simulink model "arithmetic2023"  (R2025a)
settings: Solver=FixedStepAuto  StartTime=0.0  StopTime=15  FixedStep=0.00001  MaxStep=0.001  RelTol=1e-3
values from neighbouring files (symbols this model uses):
  A = 1.5    [data2023.sldd]    (also in lqr_K.m = [0 1 0 0)
  drone_r0 = 0.0 100.0    [data.sldd]    (also in data2023.sldd = 0.0 60.0)
  Fx = 600.0    [data.sldd]    (also in data2023.sldd)
  Fy = 800.0    [data.sldd]    (also in data2023.sldd)
  g = 10.0    [data.sldd]    (also in data2023.sldd = 9.81)
  K = 3.1623 -0.0 2.7064 0.0 -0.0 3.1623 -0.0 2.7064    [data2023.sldd]    (also in lqr_K.m = lqr(A, B, Q, R))
  ma = 20.0    [data.sldd]    (also in data2023.sldd)
  mb = 50.0    [data.sldd]    (also in data2023.sldd)
  T0 = 20.0    [data.sldd]    (also in data2023.sldd)
settings Model: DataDictionary=data2023.sldd  Creator=MangoJuice  LastModifiedBy=MangoJuice

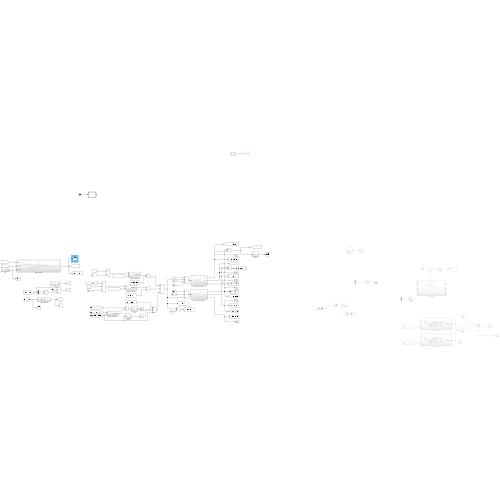
[thumbnail: Simulink's stored preview of the top-level diagram]
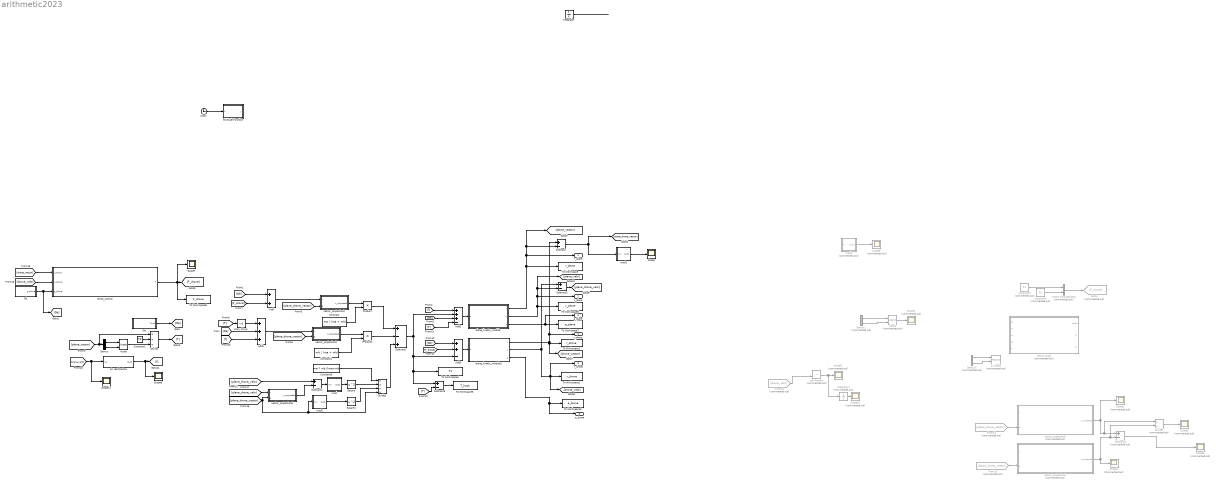
== system arithmetic2023 ==
  Add : Sum
  Add1 : Sum  Inputs=+++
  Add2 : Sum  Inputs=+++-
  Add3 : Sum  Inputs=++-
  Atan2 : Trigonometry  Commented=on  Operator=atan2
  Clock : Clock
  Constant : Constant  Value=ma / (ma + mb)
  Constant1 : Constant  Value=mb / (ma + mb)
  Constant2 : Constant  Value=T0
  Constant3 : Constant  Commented=on  Value=Fx
  Constant4 : Constant  Commented=on  Value=Fy
  Constant5 : Constant  Value=ma * mb /(ma+mb)
  Demux : Demux  Outputs=2
  Demux1 : Demux  Commented=on  Outputs=2
  Demux3 : Demux  Commented=on  Outputs=2
  Divide : Product  Inputs=**/
  Divide1 : Product  Commented=on  Inputs=*/
  Divide2 : Product  Inputs=**/*
  Dot Product : DotProduct  Commented=on  OutDataTypeStr=Inherit: Inherit via internal rule
  From13 : From  Commented=on  GotoTag=plane_drone_vector
  From14 : From  Commented=on  GotoTag=plane_drone_vector
  From20 : From  Commented=on  GotoTag=drone_velo
  Ga : Subsystem
  Gb : Subsystem
  Goto4 : Goto  Commented=on  GotoTag=F_drone
  Hypot : Math  Operator=hypot
  Integrator : Integrator
  Integrator1 : Integrator  Commented=on
  MATLAB Function : MATLAB Function  TreatAsAtomicUnit=on  SystemSampleTime=0.1
  Product : Product
  Product1 : Product
  Scope{,6..7,11} (4 alike) : Scope
      Scope settings: ActiveDisplayYMinimum=21.853261118393789  ActiveDisplayYMaximum=40.402568271734616
      Scope11 settings: ActiveDisplayYMinimum=-28.733519725359326  ActiveDisplayYMaximum=28.020670582045391  DataLoggingVariableName=ScopeData11
      Scope6 settings: ActiveDisplayYMinimum=-1  ActiveDisplayYMaximum=1  DataLoggingVariableName=ScopeData6
      Scope7 settings: ActiveDisplayYMinimum=-4257.5776928327887  ActiveDisplayYMaximum=3270.59159962983  DataLoggingVariableName=ScopeData7
  Scope{1..5,8..10} (8 alike) : Scope  Commented=on
      Scope1 settings: ActiveDisplayYMinimum=-1.0944  ActiveDisplayYMaximum=6.4337
      Scope10 settings: ActiveDisplayYMinimum=-1854.0026966671489  ActiveDisplayYMaximum=1339.365502512725  DataLoggingVariableName=ScopeData10
      Scope2 settings: ActiveDisplayYMinimum=-1  ActiveDisplayYMaximum=1  DataLoggingVariableName=ScopeData2
      Scope3 settings: ActiveDisplayYMinimum=-1.274  ActiveDisplayYMaximum=0.99186  DataLoggingVariableName=ScopeData3
      Scope4 settings: ActiveDisplayYMinimum=-0.28044128715875616  ActiveDisplayYMaximum=1.7069968813063119  DataLoggingVariableName=ScopeData4
      Scope5 settings: ActiveDisplayYMinimum=-10.224  ActiveDisplayYMaximum=15.1156  DataLoggingVariableName=ScopeData5
      Scope8 settings: ActiveDisplayYMinimum=45.49151131182159  ActiveDisplayYMaximum=877.68274656123344  DataLoggingVariableName=ScopeData8
      Scope9 settings: ActiveDisplayYMinimum=-1254.7088806848469  ActiveDisplayYMaximum=461.43323334308008  DataLoggingVariableName=ScopeData9
  Square : Math  Operator=square
  Square1 : Math  Operator=square
  Subtract{,3..5} (4 alike) : Sum  Inputs=+-
  Subtract1 : Sum  Inputs=+-+
  Subtract2 : Sum  Commented=on  Inputs=+-
  To Workspace : ToWorkspace  VariableName=r_plane  SaveFormat=Timeseries  SampleTime=0.05
  To Workspace1 : ToWorkspace  VariableName=r_drone  SaveFormat=Timeseries  SampleTime=0.05
  To Workspace2 : ToWorkspace  VariableName=v_drone  SaveFormat=Timeseries  SampleTime=0.05
  To Workspace3 : ToWorkspace  VariableName=a_drone  SaveFormat=Timeseries  SampleTime=0.05
  To Workspace4 : ToWorkspace  VariableName=T1  SaveFormat=Timeseries  SampleTime=0.05
  To Workspace5 : ToWorkspace  VariableName=T_hook  SaveFormat=Timeseries  SampleTime=0.05
  To Workspace6 : ToWorkspace  VariableName=v_plane  SaveFormat=Timeseries  SampleTime=0.05
  To Workspace7 : ToWorkspace  VariableName=a_plane  SaveFormat=Timeseries  SampleTime=0.05
  To Workspace8 : ToWorkspace  VariableName=F_drone  SaveFormat=Timeseries  SampleTime=0.05
  Unary Minus : UnaryMinus
  Vector Concatenate1 : Concatenate  Commented=on
  XY Graph : Record  Commented=on  NumPorts=2.0  FileSettingsInternal="{\"entries\":[{\"content\":{\"excelSettings\":{\"content\":{},\"type\":\"Streamout.ExcelSettings\"},\"parquetSettings\":{\"content\":{},\"type\":\"Streamout.ParquetSettings\"}},\"type\":\"Streamout.FileSettingStorage\",\"uuid\":\"\"}],\"packageUris\":[\"http:\\/\\/schema.mathworks.com\\/mf0\\/streamout_blocks\\/R2020a\"],\"version\":\"1.0\"}"  FrameSettings=[0, 0]  Layout=[1 1]  SignalsInternal="{\"entries\":[{\"content\":{\"signals\":[{\"content\":{\"blockPath\":[],\"dimensions\":[1],\"domain\":\"\",\"lineColor\":\"#a2142f\",\"plots\":[ 1 ],\"port\":1,\"signalID\":1,\"signalName\":\"Demux3:1\"},\"type\":\"RecordBlkView.Signal\",\"uuid\":\"\"},{\"content\":{\"blockPath\":[],\"dimensions\":[1],\"domain\":\"\",\"lineColor\":\"#139fff\",\"plots\":[ 1 ],\"port\":2,\"signalID\":2,\"signalName\":\"Demux3:2\"},\"type\":\"RecordBlkView.Signal\",\"uuid\":\"\"}]},\"type\":\"RecordBlkView.InputSignals\",\"uuid\":\"\"}],\"packageUris\":[\"http:\\/\\/schema.mathworks.com\\/mf0\\/streamout_blocks\\/R2020a\"],\"version\":\"1.0\"}"  VisualizationBindings="{\"xyplotplugin\":{\"info\":[{\"series\":[{\"bindingParametersList\":[{\"parameter\":\"X-Axis\",\"signalID\":1,\"signalName\":\"Demux3:1\"},{\"parameter\":\"Y-Axis\",\"signalID\":2,\"signalName\":\"Demux3:2\"}],\"seriesID\":0}],\"subplotID\":1}]}}"  CompatibilityTag=XY
  air resistantce : Subsystem
  drone_control : Subsystem
  drone_kinetic_module1 : Subsystem
  mod : Subsystem
  mod1 : Subsystem
  mod2 : Subsystem
  mod3 : Subsystem  Commented=on
  plane_kinetic_module : Subsystem
  vector-angle : Subsystem  Commented=on
  vector_projection2 : Subsystem
  vector_projection3 : Subsystem
  vector_projection4 : Subsystem  Commented=on
  vector_projection5 : Subsystem  Commented=on
  vector_projection6 : Subsystem
  r_plane : Outport
  v_plane : Outport  Port=2
  a_plane : Outport  Port=3
  r_drone : Outport  Port=4
  v_drone : Outport  Port=5
  a_drone : Outport  Port=6
  wires:
  Integrator/1 -> ?
  Ga/1(Out1) -> [Ga]
  Gb/1(g_drone) -> [Gb], drone_control/3(g_drone)
  Subtract/1 -> mod1/1(In1), [plane_drone_vector]
  Hypot/1 -> Divide/3
  [plane_vector] -> Divide/1, Demux/1
  Demux/2 -> Hypot/2
  Demux/1 -> Hypot/1
  Constant2/1 -> Divide/2
  Vector Concatenate1/1 -> Goto4/1
  Constant3/1 -> Vector Concatenate1/1
  Constant4/1 -> Vector Concatenate1/2
  [plane_drone_vector] -> vector_projection2/2(e)
  [plane_drone_vector] -> vector_projection3/2(e)
  [Gb] -> Add/1
  Product/1 -> Subtract1/1
  Product1/1 -> Subtract1/2
  Constant/1 -> Product/2
  Constant1/1 -> Product1/2
  Subtract1/1 -> Add2/2, Subtract5/1, To Workspace4/1, Add3/3
  Add2/1 -> plane_kinetic_module/1(F)
  [Ga] -> Add2/3
  [T] -> Add2/4
  Add3/1 -> drone_kinetic_module1/1(F)
  [F_drone] -> Add3/2
  [Gb] -> Add3/1
  vector_projection5/1(x_projected) -> Scope1/1, Divide1/1, Subtract2/1
  vector_projection4/1(x_projected) -> Scope2/1, Divide1/2, Subtract2/2
  From14/1 -> vector_projection5/2(e)
  From13/1 -> vector_projection4/2(e)
  Demux3/2 -> XY Graph/2
  Demux3/1 -> XY Graph/1
  Divide/1 -> [T]
  [T] -> Unary Minus/1
  Subtract2/1 -> Scope5/1
  Divide1/1 -> Scope3/1
  Subtract3/1 -> [plane_drone_velo]
  [plane_drone_velo] -> vector_projection6/1(x)
  vector_projection6/1(x_projected) -> Subtract4/2
  [plane_drone_velo] -> Subtract4/1
  Subtract4/1 -> mod/1(In1)
  mod/1(Out1) -> Square/1
  mod2/1(Out1) -> Square1/1
  [plane_drone_vector] -> vector_projection6/2(e), Divide2/4, mod2/1(In1)
  Square/1 -> Divide2/2
  Square1/1 -> Divide2/3
  Divide2/1 -> Subtract1/3
  Constant5/1 -> Divide2/1
  mod1/1(Out1) -> Scope/1
  Atan2/1 -> Scope4/1
  Demux1/1 -> Atan2/1
  Demux1/2 -> Atan2/2
  [drone_velo] -> drone_control/2(v_drone)
  [drone_vector] -> drone_control/1(r_drone)
  mod3/1(Out1) -> Scope8/1
  drone_control/1(F) -> To Workspace8/1, Scope7/1, [F_drone]
  From20/1 -> Dot Product/2
  Dot Product/1 -> Integrator1/1, Scope9/1
  Integrator1/1 -> Scope10/1
  Clock/1 -> MATLAB Function/1(t)
  [T] -> Subtract5/2
  Subtract5/1 -> To Workspace5/1
  drone_kinetic_module1/1(r) -> [drone_vector], To Workspace1/1, Subtract/1, r_drone/1
  drone_kinetic_module1/2(v) -> [drone_velo], v_drone/1, To Workspace2/1, Subtract3/1
  drone_kinetic_module1/3(a) -> a_drone/1, To Workspace3/1
  plane_kinetic_module/3(a) -> a_plane/1, To Workspace7/1
  plane_kinetic_module/2(v) -> [plane_velo], Subtract3/2, v_plane/1, To Workspace6/1
  plane_kinetic_module/1(r) -> [plane_vector], Subtract/2, r_plane/1, To Workspace/1
  [plane_velo] -> Scope11/1, air resistantce/1(In1)
  air resistantce/1(Out1) -> Scope6/1, [f]
  Unary Minus/1 -> Add1/1
  [Ga] -> Add1/2
  [f] -> Add1/3
  Add1/1 -> vector_projection3/1(x)
  vector_projection3/1(x_projected) -> Product1/1
  [F_drone] -> Add/2
  vector_projection2/1(x_projected) -> Product/1
  Add/1 -> vector_projection2/1(x)
  [f] -> Add2/1

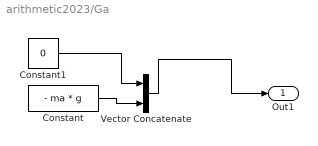
== system arithmetic2023/Ga ==
  Constant : Constant  Value=- ma * g  VectorParams1D=off
  Constant1 : Constant  Value=0
  Vector Concatenate : Concatenate
  Out1 : Outport
  wires:
  Constant1/1 -> Vector Concatenate/1
  Constant/1 -> Vector Concatenate/2
  Vector Concatenate/1 -> Out1/1

== system arithmetic2023/Gb ==
  Constant : Constant  Value=- mb * g  VectorParams1D=off
  Constant1 : Constant  Value=0
  Vector Concatenate : Concatenate
  g_drone : Outport
  wires:
  Vector Concatenate/1 -> g_drone/1
  Constant/1 -> Vector Concatenate/2
  Constant1/1 -> Vector Concatenate/1

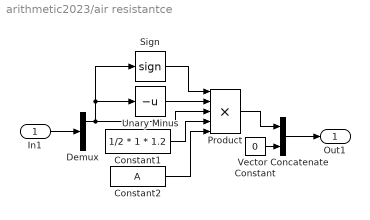
== system arithmetic2023/air resistantce ==
  In1 : Inport
  Constant : Constant  Value=0
  Constant1 : Constant  Value=1/2 * 1 * 1.2
  Constant2 : Constant  Value=A
  Demux : Demux  Outputs=2
  Product : Product  Inputs=5
  Sign : Signum
  Unary Minus : UnaryMinus
  Vector Concatenate : Concatenate
  Out1 : Outport
  wires:
  In1/1 -> Demux/1
  Demux/1 -> Product/3, Sign/1, Unary Minus/1
  Unary Minus/1 -> Product/2
  Constant1/1 -> Product/4
  Constant2/1 -> Product/5
  Product/1 -> Vector Concatenate/1
  Constant/1 -> Vector Concatenate/2
  Vector Concatenate/1 -> Out1/1
  Sign/1 -> Product/1

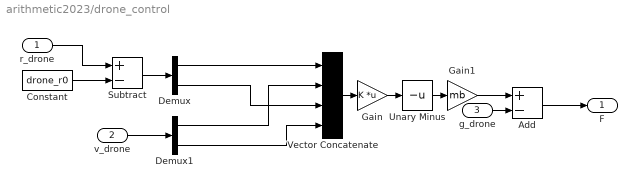
== system arithmetic2023/drone_control ==
  r_drone : Inport
  v_drone : Inport  Port=2
  g_drone : Inport  Port=3
  Add : Sum  Inputs=+-
  Constant : Constant  Value=drone_r0
  Demux : Demux  Outputs=2
  Demux1 : Demux  Outputs=2
  Gain : Gain  Gain=K  Multiplication=Matrix(K*u)
  Gain1 : Gain  Gain=mb
  Subtract : Sum  Inputs=+-
  Unary Minus : UnaryMinus
  Vector Concatenate : Concatenate  NumInputs=4
  F : Outport
  wires:
  Demux/1 -> Vector Concatenate/1
  Demux/2 -> Vector Concatenate/3
  v_drone/1 -> Demux1/1
  Demux1/2 -> Vector Concatenate/4
  Demux1/1 -> Vector Concatenate/2
  Vector Concatenate/1 -> Gain/1
  Unary Minus/1 -> Gain1/1
  Gain/1 -> Unary Minus/1
  Add/1 -> F/1
  Subtract/1 -> Demux/1
  r_drone/1 -> Subtract/1
  Constant/1 -> Subtract/2
  g_drone/1 -> Add/2
  Gain1/1 -> Add/1

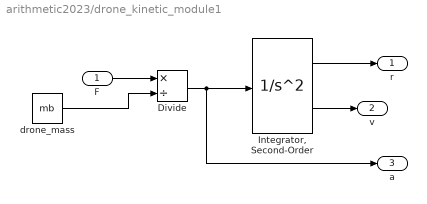
== system arithmetic2023/drone_kinetic_module1 ==
  F : Inport
  Divide : Product  Inputs=*/
  "Integrator, Second-Order" : SecondOrderIntegrator  ICX=drone_r0  ICDXDT=drone_v0
  drone_mass : Constant  Value=mb
  r : Outport
  v : Outport  Port=2
  a : Outport  Port=3
  wires:
  drone_mass/1 -> Divide/2
  "Integrator, Second-Order"/2 -> v/1
  "Integrator, Second-Order"/1 -> r/1
  Divide/1 -> a/1, "Integrator, Second-Order"/1
  F/1 -> Divide/1

== system arithmetic2023/mod ==
  In1 : Inport
  Demux4 : Demux  Outputs=2
  Hypot3 : Math  Operator=hypot
  Out1 : Outport
  wires:
  Demux4/1 -> Hypot3/1
  Demux4/2 -> Hypot3/2
  In1/1 -> Demux4/1
  Hypot3/1 -> Out1/1

== system arithmetic2023/mod1 ==
  In1 : Inport
  Demux4 : Demux  Outputs=2
  Hypot3 : Math  Operator=hypot
  Out1 : Outport
  wires:
  Demux4/1 -> Hypot3/1
  Demux4/2 -> Hypot3/2
  In1/1 -> Demux4/1
  Hypot3/1 -> Out1/1

== system arithmetic2023/mod2 ==
  In1 : Inport
  Demux4 : Demux  Outputs=2
  Hypot3 : Math  Operator=hypot
  Out1 : Outport
  wires:
  Hypot3/1 -> Out1/1
  In1/1 -> Demux4/1
  Demux4/2 -> Hypot3/2
  Demux4/1 -> Hypot3/1

== system arithmetic2023/mod3 ==
  F : Inport
  Demux4 : Demux  Outputs=2
  Hypot3 : Math  Operator=hypot
  Out1 : Outport
  wires:
  Hypot3/1 -> Out1/1
  F/1 -> Demux4/1
  Demux4/2 -> Hypot3/2
  Demux4/1 -> Hypot3/1

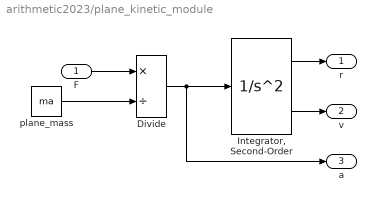
== system arithmetic2023/plane_kinetic_module ==
  F : Inport
  Divide : Product  Inputs=*/
  "Integrator, Second-Order" : SecondOrderIntegrator  ICX=plane_r0  ICDXDT=plane_v0
  plane_mass : Constant  Value=ma
  r : Outport
  v : Outport  Port=2
  a : Outport  Port=3
  wires:
  F/1 -> Divide/1
  Divide/1 -> "Integrator, Second-Order"/1, a/1
  "Integrator, Second-Order"/1 -> r/1
  "Integrator, Second-Order"/2 -> v/1
  plane_mass/1 -> Divide/2

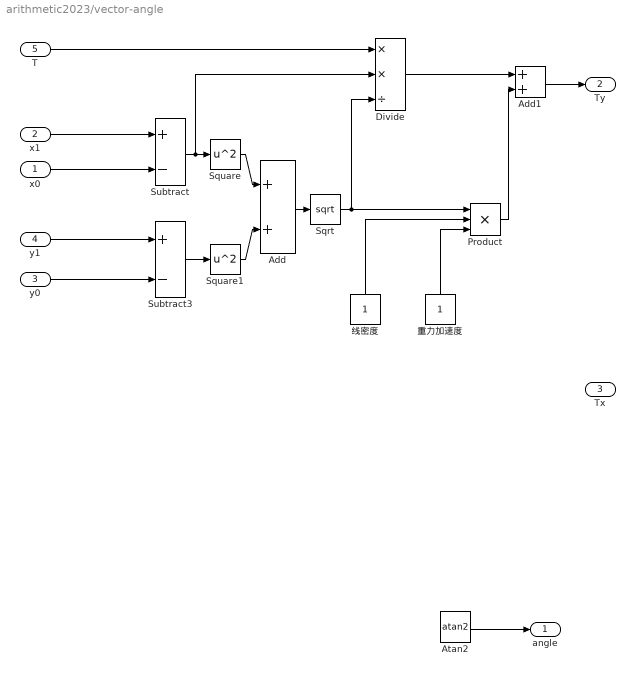
== system arithmetic2023/vector-angle ==
  x0 : Inport
  x1 : Inport  Port=2
  y0 : Inport  Port=3
  y1 : Inport  Port=4
  T : Inport  Port=5
  Add : Sum
  Add1 : Sum
  Atan2 : Trigonometry  Operator=atan2
  Divide : Product  Inputs=**/
  Product : Product  Inputs=3
  Sqrt : Sqrt
  Square : Math  Operator=square
  Square1 : Math  Operator=square
  Subtract : Sum  Inputs=+-
  Subtract3 : Sum  Inputs=+-
  线密度 : Constant
  重力加速度 : Constant
  angle : Outport
  Ty : Outport  Port=2
  Tx : Outport  Port=3
  wires:
  y0/1 -> Subtract3/2
  x1/1 -> Subtract/1
  Atan2/1 -> angle/1
  x0/1 -> Subtract/2
  y1/1 -> Subtract3/1
  Subtract/1 -> Divide/2, Square/1
  Subtract3/1 -> Square1/1
  Square/1 -> Add/1
  Square1/1 -> Add/2
  线密度/1 -> Product/2
  重力加速度/1 -> Product/3
  T/1 -> Divide/1
  Add/1 -> Sqrt/1
  Sqrt/1 -> Divide/3, Product/1
  Divide/1 -> Add1/1
  Product/1 -> Add1/2
  Add1/1 -> Ty/1

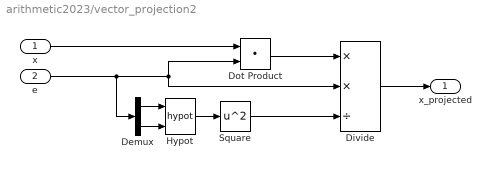
== system arithmetic2023/vector_projection2 ==
  x : Inport
  e : Inport  Port=2
  Demux : Demux  Outputs=2
  Divide : Product  Inputs=**/
  Dot Product : DotProduct  OutDataTypeStr=Inherit: Inherit via internal rule
  Hypot : Math  Operator=hypot
  Square : Math  Operator=square
  x_projected : Outport
  wires:
  x/1 -> Dot Product/1
  Divide/1 -> x_projected/1
  Hypot/1 -> Square/1
  e/1 -> Demux/1, Dot Product/2, Divide/2
  Demux/2 -> Hypot/2
  Demux/1 -> Hypot/1
  Square/1 -> Divide/3
  Dot Product/1 -> Divide/1

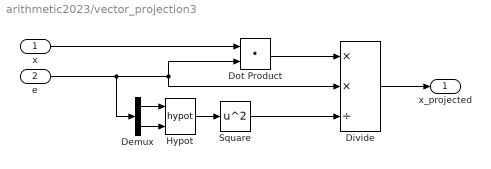
== system arithmetic2023/vector_projection3 ==
  x : Inport
  e : Inport  Port=2
  Demux : Demux  Outputs=2
  Divide : Product  Inputs=**/
  Dot Product : DotProduct  OutDataTypeStr=Inherit: Inherit via internal rule
  Hypot : Math  Operator=hypot
  Square : Math  Operator=square
  x_projected : Outport
  wires:
  Dot Product/1 -> Divide/1
  Square/1 -> Divide/3
  Demux/1 -> Hypot/1
  Demux/2 -> Hypot/2
  e/1 -> Divide/2, Dot Product/2, Demux/1
  Hypot/1 -> Square/1
  Divide/1 -> x_projected/1
  x/1 -> Dot Product/1

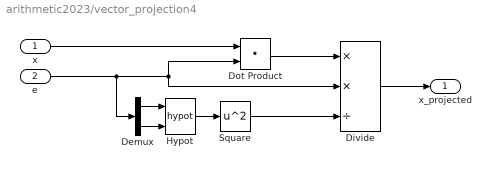
== system arithmetic2023/vector_projection4 ==
  x : Inport
  e : Inport  Port=2
  Demux : Demux  Outputs=2
  Divide : Product  Inputs=**/
  Dot Product : DotProduct  OutDataTypeStr=Inherit: Inherit via internal rule
  Hypot : Math  Operator=hypot
  Square : Math  Operator=square
  x_projected : Outport
  wires:
  Dot Product/1 -> Divide/1
  Square/1 -> Divide/3
  Demux/1 -> Hypot/1
  Demux/2 -> Hypot/2
  e/1 -> Divide/2, Dot Product/2, Demux/1
  Hypot/1 -> Square/1
  Divide/1 -> x_projected/1
  x/1 -> Dot Product/1

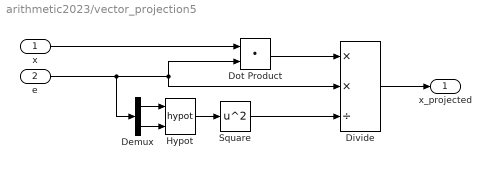
== system arithmetic2023/vector_projection5 ==
  x : Inport
  e : Inport  Port=2
  Demux : Demux  Outputs=2
  Divide : Product  Inputs=**/
  Dot Product : DotProduct  OutDataTypeStr=Inherit: Inherit via internal rule
  Hypot : Math  Operator=hypot
  Square : Math  Operator=square
  x_projected : Outport
  wires:
  x/1 -> Dot Product/1
  Divide/1 -> x_projected/1
  Hypot/1 -> Square/1
  e/1 -> Demux/1, Dot Product/2, Divide/2
  Demux/2 -> Hypot/2
  Demux/1 -> Hypot/1
  Square/1 -> Divide/3
  Dot Product/1 -> Divide/1

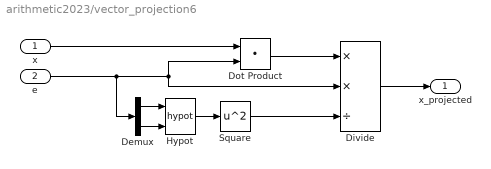
== system arithmetic2023/vector_projection6 ==
  x : Inport
  e : Inport  Port=2
  Demux : Demux  Outputs=2
  Divide : Product  Inputs=**/
  Dot Product : DotProduct  OutDataTypeStr=Inherit: Inherit via internal rule
  Hypot : Math  Operator=hypot
  Square : Math  Operator=square
  x_projected : Outport
  wires:
  Dot Product/1 -> Divide/1
  Square/1 -> Divide/3
  Demux/1 -> Hypot/1
  Demux/2 -> Hypot/2
  e/1 -> Divide/2, Dot Product/2, Demux/1
  Hypot/1 -> Square/1
  Divide/1 -> x_projected/1
  x/1 -> Dot Product/1

== matlab function arithmetic2023/MATLAB Function ==
  data: t input; y output
function y = show_time(t)
y = 0;  
persistent target
if isempty(target)
    target = 0.0;
end

if abs(target - t) < 1e-3  % 每2s打印一次
    fprintf('Sim Time: %.2fs\n', t);
    target = target + 2;
end
